simulink model "tpauto6"  (R2019a)
settings: Solver=VariableStepAuto  StartTime=0.0  StopTime=10.0  RelTol=1e-3
undefined symbols (not defined in the file): alpha0, alphapoint0, g, l
settings Model: Creator=mbenahme  LastModifiedBy=mbenahme

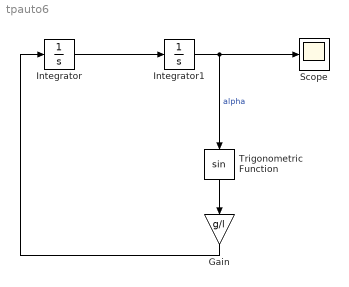
== system tpauto6 ==
  Gain : Gain  Gain=g/l
  Integrator : Integrator  InitialCondition=alphapoint0
  Integrator1 : Integrator  InitialCondition=alpha0
  Scope : Scope
  Trigonometric Function : Trigonometry
  wires:
  Integrator/1 -> Integrator1/1
  Integrator1/1 -> Scope/1, Trigonometric Function/1  "alpha"
  Trigonometric Function/1 -> Gain/1
  Gain/1 -> Integrator/1
